simulink model "StNumChk"  (R2018b)
settings: Solver=FixedStepDiscrete  StartTime=0.0  StopTime=10.0  FixedStep=0.01  RelTol=1e-3
undefined symbols (not defined in the file or in its folder): IfVeSMSeStNumConfig
settings Model: Creator=sn2xws  LastModifiedBy=sn2xws
settings DataIOCC: SaveFormat=StructureWithTime
settings OptimizationCC: DefaultParameterBehavior=Inlined  EnhancedBackFolding=on  PassReuseOutputArgsAs=Individual arguments  ZeroExternalMemoryAtStartup=off  ZeroInternalMemoryAtStartup=off  OptimizeBlockOrder=speed  DifferentSizesBufferReuse=on  OptimizationCustomize=off
settings DebuggingCC: ParameterTunabilityLossMsg=error
settings ModelReferenceCC: ModelReferenceNumInstancesAllowed=Single
settings SFSimCC: MATLABDynamicMemAlloc=off
settings RTWCC: SystemTargetFile=autosar.tlc  GenCodeOnly=on  TemplateMakefile=ert_default_tmf  Description=AUTOSAR  GenerateReport=on  IncludeHyperlinkInReport=on  LaunchReport=on  GenerateTraceInfo=on  GenerateTraceReport=on  GenerateTraceReportSl=on  GenerateTraceReportSf=on  GenerateTraceReportEml=on
settings CodeAppCC: ForceParamTrailComments=on  IgnoreCustomStorageClasses=off  OperatorAnnotations=on  SimulinkDataObjDesc=on  SFDataObjDesc=on  InsertBlockDesc=on
settings STFCustomTargetCC: TargetLangStandard=C99 (ISO)  MultiwordLength=256  ParMdlRefBuildCompliant=on  CompOptLevelCompliant=on  IncludeMdlTerminateFcn=off  CombineOutputUpdateFcns=on  SuppressErrorStatus=on  ERTCustomFileBanners=on  SupportNonFinite=off  SupportComplex=off  SupportContinuousTime=off  SupportNonInlinedSFcns=off  RemoveResetFunc=on  MATLABClassNameForMDSCustomization=Simulink.SoftwareTarget.ERTCustomization  AutosarCompliant=on  UseToolchainInfoCompliant=on  LookupTableObjectStructAxisOrder=2,1,3,4,...  LUTObjectStructOrderEvenSpacing=Size,Table,Breakpoints  SystemTargetFile=autosar.tlc
settings ERTTargetCC: TargetLangStandard=C99 (ISO)  ConcurrentExecutionCompliant=off  IncludeMdlTerminateFcn=off  SuppressErrorStatus=on  SupportNonFinite=off  SupportComplex=off  ModelStepFunctionPrototypeControlCompliant=off  CPPClassGenCompliant=off  AutosarCompliant=on  LookupTableObjectStructAxisOrder=2,1,3,4,...  LUTObjectStructOrderEvenSpacing=Size,Table,Breakpoints  InlinedParameterPlacement=NonHierarchical  ERTCustomFileTemplate=example_file_process.tlc  ERTFilePackagingFormat=Compact

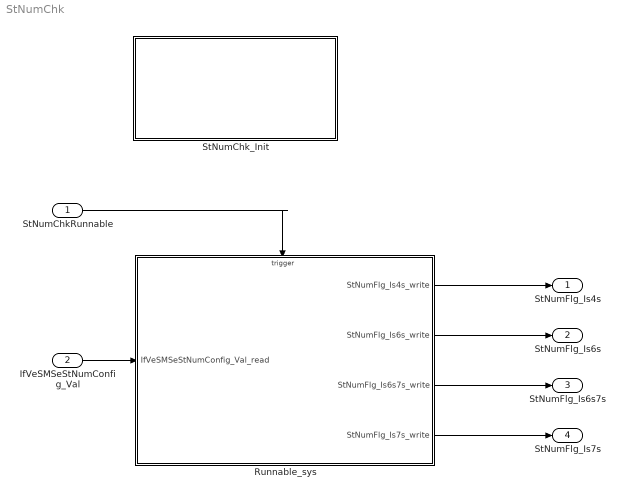
== system StNumChk ==
  StNumChkRunnable : Inport  SampleTime=0.01  OutputFunctionCall=on
  IfVeSMSeStNumConfig_Val : Inport  Port=2  OutDataTypeStr=Enum: IfVeSMSeStNumConfig  PortDimensions=1
  Runnable_sys : Subsystem
  StNumChk_Init : Subsystem
  StNumFlg_Is4s : Outport  OutDataTypeStr=boolean  PortDimensions=1
  StNumFlg_Is6s : Outport  Port=2  OutDataTypeStr=boolean  PortDimensions=1
  StNumFlg_Is6s7s : Outport  Port=3  OutDataTypeStr=boolean  PortDimensions=1
  StNumFlg_Is7s : Outport  Port=4  OutDataTypeStr=boolean  PortDimensions=1
  wires:
  IfVeSMSeStNumConfig_Val/1 -> Runnable_sys/1(IfVeSMSeStNumConfig_Val_read)
  Runnable_sys/1(StNumFlg_Is4s_write) -> StNumFlg_Is4s/1
  Runnable_sys/2(StNumFlg_Is6s_write) -> StNumFlg_Is6s/1
  Runnable_sys/3(StNumFlg_Is6s7s_write) -> StNumFlg_Is6s7s/1
  Runnable_sys/4(StNumFlg_Is7s_write) -> StNumFlg_Is7s/1
  StNumChkRunnable/1 -> Runnable_sys/Trigger

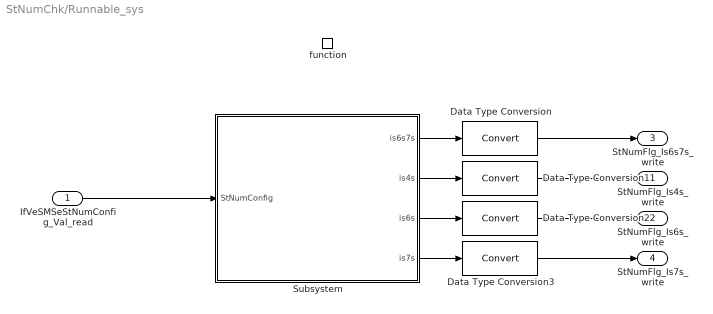
== system StNumChk/Runnable_sys ==
  IfVeSMSeStNumConfig_Val_read : Inport
  function : TriggerPort  TriggerType=function-call  VariantControl=(inherit)
  Data Type Conversion{,1..3} (4 alike) : DataTypeConversion
  Subsystem : Subsystem
  StNumFlg_Is4s_write : Outport
      settings: EnsureOutportIsVirtual=on
  StNumFlg_Is6s_write : Outport  Port=2
      settings: EnsureOutportIsVirtual=on
  StNumFlg_Is6s7s_write : Outport  Port=3
      settings: EnsureOutportIsVirtual=on
  StNumFlg_Is7s_write : Outport  Port=4
      settings: EnsureOutportIsVirtual=on
  wires:
  IfVeSMSeStNumConfig_Val_read/1 -> Subsystem/1(StNumConfig)
  Subsystem/2(is4s) -> Data Type Conversion1/1
  Subsystem/3(is6s) -> Data Type Conversion2/1
  Subsystem/1(is6s7s) -> Data Type Conversion/1
  Subsystem/4(is7s) -> Data Type Conversion3/1
  Data Type Conversion/1 -> StNumFlg_Is6s7s_write/1
  Data Type Conversion1/1 -> StNumFlg_Is4s_write/1
  Data Type Conversion2/1 -> StNumFlg_Is6s_write/1
  Data Type Conversion3/1 -> StNumFlg_Is7s_write/1

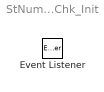
== system StNumChk/StNumChk_Init ==
  Event Listener : EventListener  EventName=reset

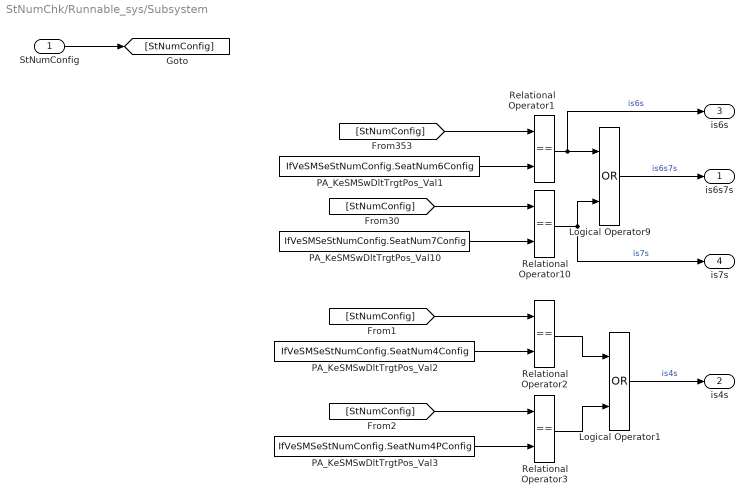
== system StNumChk/Runnable_sys/Subsystem ==
  StNumConfig : Inport
  Logical Operator1 : Logic  Operator=OR  AllPortsSameDT=off  OutDataTypeStr=boolean
  Logical Operator9 : Logic  Operator=OR  AllPortsSameDT=off  OutDataTypeStr=boolean
  PA_KeSMSwDltTrgtPos_Val1 : Constant  Value=IfVeSMSeStNumConfig.SeatNum6Config  OutDataTypeStr=Enum:IfVeSMSeStNumConfig
  PA_KeSMSwDltTrgtPos_Val10 : Constant  Value=IfVeSMSeStNumConfig.SeatNum7Config  OutDataTypeStr=Enum:IfVeSMSeStNumConfig
  PA_KeSMSwDltTrgtPos_Val2 : Constant  Value=IfVeSMSeStNumConfig.SeatNum4Config  OutDataTypeStr=Enum:IfVeSMSeStNumConfig
  PA_KeSMSwDltTrgtPos_Val3 : Constant  Value=IfVeSMSeStNumConfig.SeatNum4PConfig  OutDataTypeStr=Enum:IfVeSMSeStNumConfig
  Relational Operator{1..3,10} (4 alike) : RelationalOperator  Operator===  OutDataTypeStr=boolean  RndMeth=Simplest
  is6s7s : Outport
  is4s : Outport  Port=2
  is6s : Outport  Port=3
  is7s : Outport  Port=4
  wires:
  Relational Operator1/1 -> is6s/1, Logical Operator9/1  "is6s"
  Logical Operator9/1 -> is6s7s/1  "is6s7s"
  [StNumConfig] -> Relational Operator1/1
  [StNumConfig] -> Relational Operator10/1
  PA_KeSMSwDltTrgtPos_Val1/1 -> Relational Operator1/2
  Relational Operator10/1 -> is7s/1, Logical Operator9/2  "is7s"
  PA_KeSMSwDltTrgtPos_Val10/1 -> Relational Operator10/2
  StNumConfig/1 -> [StNumConfig]
  [StNumConfig] -> Relational Operator2/1
  PA_KeSMSwDltTrgtPos_Val2/1 -> Relational Operator2/2
  [StNumConfig] -> Relational Operator3/1
  PA_KeSMSwDltTrgtPos_Val3/1 -> Relational Operator3/2
  Relational Operator2/1 -> Logical Operator1/1
  Relational Operator3/1 -> Logical Operator1/2
  Logical Operator1/1 -> is4s/1  "is4s"
